simulink subsystem "Battery"  (R2025b)
settings: Solver=VariableStepAuto  StartTime=0.0  StopTime=10.0  RelTol=1e-3
values from neighbouring files (symbols this model uses):
  C_init = C_total*.8    (= 259200)    [Parameters_Buck.m]
  C_total = 90 * 3600    (= 324000)    [Parameters_Buck.m]
  P01A = [42.2942  -98.3961   88.7769  -40.3893   10.2942   11.4802]    [Parameters_Buck.m]
  Rbat = 21.6e-3*4    (= 0.0864)    [Parameters_Buck.m]
settings Model: Creator=carter  LastModifiedBy=carter

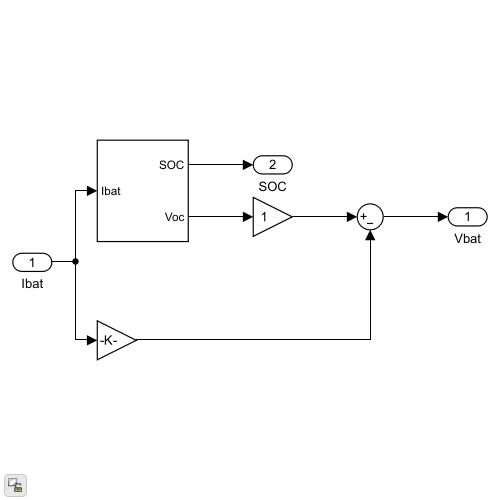
[thumbnail: Simulink's stored preview of the top-level diagram]
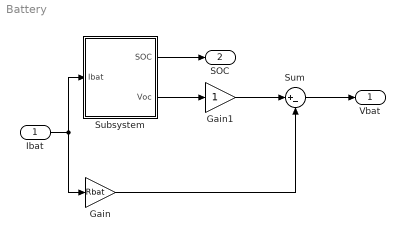
== system Battery ==
  Ibat : Inport
  Gain : Gain  Gain=Rbat
  Gain1 : Gain
  Subsystem : Subsystem
  Sum : Sum  Inputs=|+-
  Vbat : Outport
  SOC : Outport  Port=2
  wires:
  Ibat/1 -> Subsystem/1(Ibat), Gain/1
  Gain/1 -> Sum/2
  Sum/1 -> Vbat/1
  Gain1/1 -> Sum/1
  Subsystem/2(Voc) -> Gain1/1
  Subsystem/1(SOC) -> SOC/1

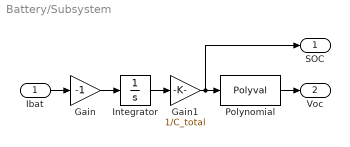
== system Battery/Subsystem ==
  Ibat : Inport
  Gain : Gain  Gain=-1
  Gain1 : Gain  Gain=1/C_total
  Integrator : Integrator  InitialCondition=C_init  LimitOutput=on  UpperSaturationLimit=C_total  LowerSaturationLimit=0
  Polynomial : Polyval  Coefs=P01A
  SOC : Outport
  Voc : Outport  Port=2
  wires:
  Polynomial/1 -> Voc/1
  Gain1/1 -> Polynomial/1, SOC/1
  Integrator/1 -> Gain1/1
  Gain/1 -> Integrator/1
  Ibat/1 -> Gain/1
